simulink model "q5"  (R2021b)
settings: Solver=VariableStepAuto  StartTime=0.0  StopTime=10.0  RelTol=1e-3
settings Model: Creator=Arthur  LastModifiedBy=Arthur
settings DataIOCC: SaveFormat=Array

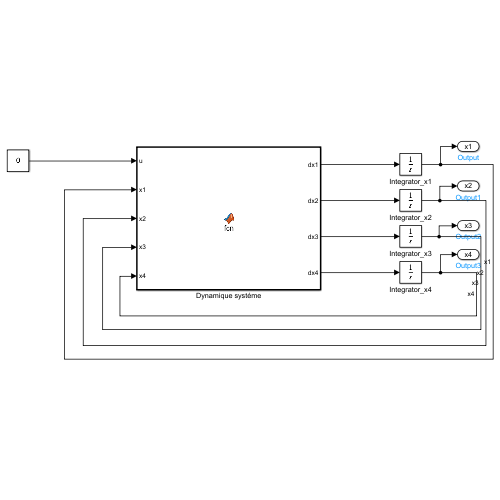
[thumbnail: Simulink's stored preview of the top-level diagram]
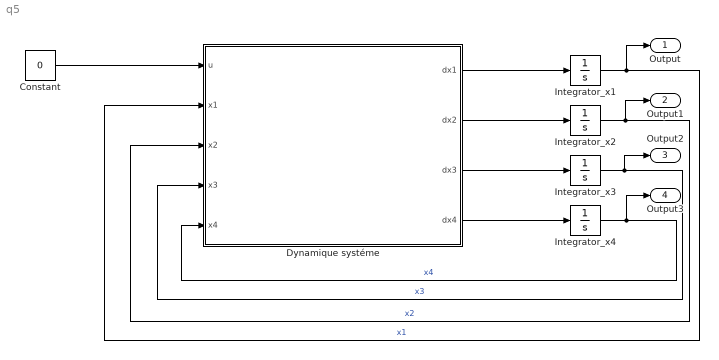
== system q5 ==
  Constant : Constant  Value=0
  Dynamique systéme : MATLAB Function  TreatAsAtomicUnit=on
  Integrator_x{1..4} (4 alike) : Integrator
  Output : Outport
  Output1 : Outport  Port=2
  Output2 : Outport  Port=3
  Output3 : Outport  Port=4
  wires:
  Dynamique systéme/1(dx1) -> Integrator_x1/1
  Dynamique systéme/2(dx2) -> Integrator_x2/1
  Dynamique systéme/3(dx3) -> Integrator_x3/1
  Dynamique systéme/4(dx4) -> Integrator_x4/1
  Integrator_x4/1 -> Output3/1, Dynamique systéme/5(x4)  "x4"
  Integrator_x3/1 -> Dynamique systéme/4(x3), Output2/1  "x3"
  Integrator_x2/1 -> Dynamique systéme/3(x2), Output1/1  "x2"
  Integrator_x1/1 -> Dynamique systéme/2(x1), Output/1  "x1"
  Constant/1 -> Dynamique systéme/1(u)

== matlab function q5/Dynamique systéme ==
  data: u input; dx1 output; x1 input; x2 input; x3 input; x4 input; dx2 output; dx3 output; dx4 output
function [dx1,dx2,dx3,dx4] = fcn(u,x1,x2,x3,x4)
    % declaration constants
    J = 0.02; % kg.m^2
    m = 0.6; % kg
    sigma = 0.8; % adimentional
    g = 9.81; % m/s^2
    
    % dynamique
    dx1 = x2;
    dx2 = (x1*x4*x4-g*sin(x3))/(1+sigma);
    dx3 = x4;
    dx4 = (u-m*g*x1*cos(x3)-2*m*x1*x2*x4)/(J+m*x1*x1);
